simulink model "Assembly_Throwing_Arm"  (R2021a)
settings: Solver=ode15s  StartTime=0.0  StopTime=0.09
InitFcn:
  | contact_stiffness = 2000;
  | contact_damping = 10;
  | 
  | %% Parameters
  | 
  | %------------------- Mechanical -------------------%
  | arm_len = 0.106;
  | launch_ang = 45*(pi/180);
  | th_start = 0;
  | r_ball = 31.5/1000;
  | g = -9.80665;
  | 
  | %------------------- Electrical -------------------%
  | R = 0.194;
  | L = 0.097*1e-3;
  | K_m = 1/24.48;
  | V_max = 24;
  | neta = 0.70;
  | n = 6.5;
  | f_s = 4000;
  | NL_speed = 1200;
  | R_speed = 1050;
  | R_power = 240;
  | NL_current = 0.98;
  | 
  | 
  | %NL_speed = 589;
  | %R_speed = 469;
  | %R_power = 24*15.7;
  | %NL_current = 0.98;
model workspace: external: MATLAB File C:\Users\Imad\Downloads\Throwing Arm 3\Assembly_Throwing_Arm_DataFile.m (data not in the file)
values from neighbouring files (symbols this model uses):
  smiData = struct    [Assembly_Throwing_Arm_DataFile.m]
  target = target_given(1,3)    [Script_Throwing_Arm.m]
undefined symbols (not defined in the file or in its folder): X, Y, Z
libraries: sm_lib x20, nesl_utility x9, fl_lib x8, ee_lib x3, pid_lib x2
(part 1 of 2)
settings Model: OrderedModelArguments=off  Creator=Imad  LastModifiedBy=Imad
settings SolverCC: ZeroCrossControl=DisableAll

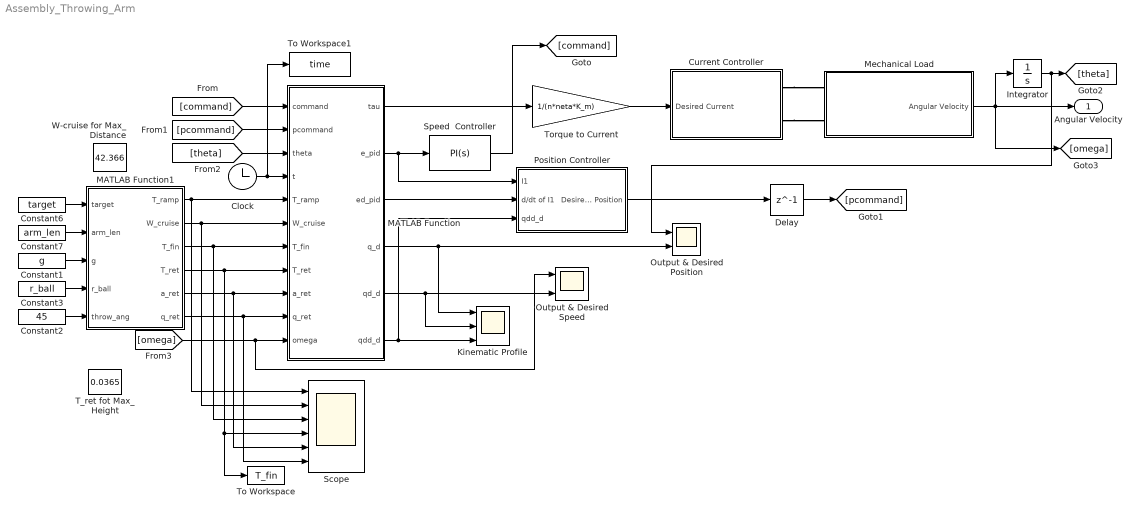
== system Assembly_Throwing_Arm ==
  Clock : Clock
  Constant1 : Constant  Value=g
  Constant2 : Constant  Value=45
  Constant3 : Constant  Value=r_ball
  Constant6 : Constant  Value=target
  Constant7 : Constant  Value=arm_len
  Current Controller : Subsystem
  Delay : Delay  DelayLength=1  SampleTime=1/(1*f_s)
  Integrator : Integrator
  Kinematic Profile : Scope  NumInputPorts=3
  MATLAB Function : MATLAB Function  TreatAsAtomicUnit=on
  MATLAB Function1 : MATLAB Function  TreatAsAtomicUnit=on
  Mechanical Load : Subsystem
  Output & Desired Position : Scope  NumInputPorts=2
  Output & Desired Speed : Scope  NumInputPorts=2
  "Position Controller " : Subsystem
  Scope : Scope  NumInputPorts=6
  Speed  Controller : pid_lib/PID Controller  Controller=PI  Form=Parallel  TimeDomain=Continuous-time  UseExternalTs=off  SampleTime=1/4000  IntegratorMethod=Forward Euler  FilterMethod=Forward Euler  ControllerParametersSource=internal  P=970*L*9  I=135*R  D=-0.5  UseFilter=on  N=100  TunerSelectOption=Frequency Response Based  InitialConditionSource=internal  InitialConditionForIntegrator=0  InitialConditionForFilter=0  DifferentiatorICPrevScaledInput=0  ExternalReset=none  TrackingMode=off  Kt=1  LimitOutput=off  SatLimitsSource=internal  UpperSaturationLimit=inf  LowerSaturationLimit=-inf  LinearizeAsGain=on  AntiWindupMode=none  Kb=1  POutMin=[]  POutMax=[]  IOutMin=[]  IOutMax=[]  DOutMin=[]  DOutMax=[]  NOutMin=[]  NOutMax=[]  SumOutMin=[]  SumOutMax=[]  SaturationOutMin=[]  SaturationOutMax=[]  PParamMin=[]  PParamMax=[]  IParamMin=[]  IParamMax=[]  DParamMin=[]  DParamMax=[]  NParamMin=[]  NParamMax=[]  KbParamMin=[]  KbParamMax=[]  KtParamMin=[]  KtParamMax=[]  KbOutMin=[]  KbOutMax=[]  KtOutMin=[]  KtOutMax=[]  IntegratorOutMin=[]  IntegratorOutMax=[]  FilterOutMin=[]  FilterOutMax=[]  SumI1OutMin=[]  SumI1OutMax=[]  SumI2OutMin=[]  SumI2OutMax=[]  SumI3OutMin=[]  SumI3OutMax=[]  SumI4OutMin=[]  SumI4OutMax=[]  SumDOutMin=[]  SumDOutMax=[]  DifferentiatorOutMin=[]  DifferentiatorOutMax=[]  FilterDiffOutCoefMin=[]  FilterDiffOutCoefMax=[]  ReciprocalOutMin=[]  ReciprocalOutMax=[]  SumDenOutMin=[]  SumDenOutMax=[]  SumNumOutMin=[]  SumNumOutMax=[]  DivideOutMin=[]  DivideOutMax=[]  UdiffTsProdOutMin=[]  UdiffTsProdOutMax=[]  NTsProdOutMin=[]  NTsProdOutMax=[]  UintegralTsProdOutMin=[]  UintegralTsProdOutMax=[]  UngainTsProdOutMin=[]  UngainTsProdOutMax=[]  IntegratorContinuousStateAttributes=''  IntegratorStateMustResolveToSignalObject=off  IntegratorRTWStateStorageClass=Auto  FilterContinuousStateAttributes=''  FilterStateMustResolveToSignalObject=off  FilterRTWStateStorageClass=Auto  ParallelPVariant=InternalParameters  IdealPVariant=Disabled  IVariant=InternalParameters  DVariant=Disabled  IntegratorVariant=Continuous  SatVariant=Disabled  AWVariant=Passthrough  PCopyVariant=Disabled  TRVariant=Disabled  FdbkBlocksVariant=Forward  IdealPFdbkVariant=Disabled  SatFdbkVariant=Disabled  DerivativeFilterVariant=Disabled  NVariant=Disabled  NCopyVariant=Disabled_SignalSpec  FilterICVariant=Disabled  IntegratorICVariant=InternalICs  ExternalResetVariant=Disabled  TRSumVariant=Passthrough  SumFdbkVariant=Disabled  SumVariant=Sum_PI  TsampFilterVariant=InternalTs  TsampNgainVariant=Passthrough  TsampIntegralVariant=Passthrough  ExternalSaturationOutDataTypeStr=Inherit: Same as second input
  T_ret fot Max_Height : Constant  Value=0.0365
  To Workspace : ToWorkspace  VariableName=T_fin  SampleTime=-1
      settings: Save2DSignal=2-D array (concatenate along first dimension)
  To Workspace1 : ToWorkspace  VariableName=time  SampleTime=-1
  Torque to Current : Gain  Gain=1/(n*neta*K_m)
  W-cruise for Max_Distance : Constant  Value=42.366
  Angular Velocity : Outport
  wires:
  MATLAB Function/3(ed_pid) -> "Position Controller "/2(d/dt of I1)
  MATLAB Function/6(qdd_d) -> Kinematic Profile/3, "Position Controller "/3(qdd_d)
  Clock/1 -> To Workspace1/1, MATLAB Function/4(t)
  [command] -> MATLAB Function/1(command)
  [pcommand] -> MATLAB Function/2(pcommand)
  Torque to Current/1 -> Current Controller/1("Desired Current ")
  Mechanical Load/1(Angular Velocity) -> Integrator/1, Angular Velocity/1, [omega]
  Delay/1 -> [pcommand]
  [theta] -> MATLAB Function/3(theta)
  Speed  Controller/1 -> [command]
  MATLAB Function1/1(T_ramp) -> Scope/1, MATLAB Function/5(T_ramp)
  MATLAB Function1/2(W_cruise) -> MATLAB Function/6(W_cruise), Scope/2
  MATLAB Function1/3(T_fin) -> Scope/3, MATLAB Function/7(T_fin)
  MATLAB Function1/4(T_ret) -> MATLAB Function/8(T_ret), Scope/4, To Workspace/1
  MATLAB Function/2(e_pid) -> Speed  Controller/1, "Position Controller "/1(I1)
  Constant7/1 -> MATLAB Function1/2(arm_len)
  Constant6/1 -> MATLAB Function1/1(target)
  Constant2/1 -> MATLAB Function1/5(throw_ang)
  Constant1/1 -> MATLAB Function1/3(g)
  MATLAB Function1/5(a_ret) -> MATLAB Function/9(a_ret), Scope/5
  MATLAB Function1/6(q_ret) -> MATLAB Function/10(q_ret), Scope/6
  "Position Controller "/1(Desired Position) -> Delay/1
  MATLAB Function/1(tau) -> Torque to Current/1
  Constant3/1 -> MATLAB Function1/4(r_ball)
  Integrator/1 -> Output & Desired Position/1, [theta]
  MATLAB Function/4(q_d) -> Output & Desired Position/2, Kinematic Profile/1
  [omega] -> Output & Desired Speed/1, MATLAB Function/11(omega)
  MATLAB Function/5(qd_d) -> Output & Desired Speed/2, Kinematic Profile/2
  connections:
  Current Controller/RConn1 -- Mechanical Load/LConn1
  Current Controller/RConn2 -- Mechanical Load/LConn2

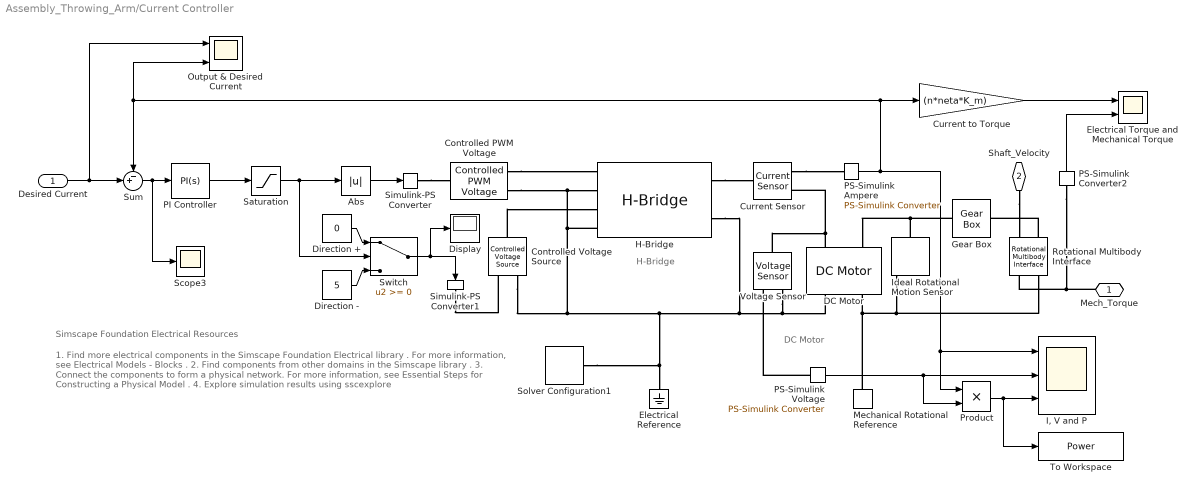
== system Assembly_Throwing_Arm/Current Controller ==
  note: H-Bridge
  note: DC Motor
  note: 1. Find more electrical components in the Simscape Foundation Electrical library .
      | For more information, see Electrical Models - Blocks .
      | 2. Find components from other domains in the Simscape library .
      | 3. Connect the components to form a physical network.
      | For more information, see Essential Steps for Constructing a Physical Model .
      | 4. Explore simulation results using sscexplore
  note: Simscape Foundation Electrical Resources
  "Desired Current " : Inport
  Abs : Abs
  Controlled PWM Voltage : ee_lib/Integrated Circuits/Controlled PWM Voltage  F=f_s Hz  TD=0 s  pulse_width_offset=0 s  pulse_min=1 us  Vmin=0 V  Vmax=12 V  Vm=V_max V  pwm_or_av=2  event_type=1  sample_time=1e-6 s  u_min=0  u_max=V_max
      settings: InternalSimscapePortConfiguration="{\"Bottom\":[],\"Left\":[{\"id\":\"u\",\"label\":\"u\",\"type\":\"input\"}],\"Right\":[{\"id\":\"p2\",\"label\":\"PWM\",\"type\":\"foundation.electrical.electrical\"},{\"id\":\"n2\",\"label\":\"REF\",\"type\":\"foundation.electrical.electrical\"}],\"Top\":[]}"
  Controlled Voltage Source : fl_lib/Electrical/Electrical Sources/Controlled Voltage Source
  Current Sensor : fl_lib/Electrical/Electrical Sensors/Current Sensor
  Current to Torque : Gain  Gain=(n*neta*K_m)
  DC Motor : ee_lib/Electromechanical/Brushed Motors/DC Motor  field_option=ee.enum.field_option.pm  Rf=100 Ohm  Lf=1 H  Laf=0.15 H  If0=0 A  parameterization=ee.enum.dcparam_option.load_speed  Ra=R Ohm  La=L H  emf_or_torque=ee.enum.emf_or_torque.kv  Kv=K_m V/rpm  Ki=6.876e-4 N*m/A  T_stall=4.5 N*m  w_max=NL_speed rpm  w_rated=R_speed rpm  P_rated=R_power W  V_rated=V_max V  J=2000 g*cm^2  lam_param=ee.enum.lam_param.current  lam=(1.114e-4) N*m/(rad/s)  i_noload=NL_current A  V_i_noload=V_max V  speed0=0 rpm  enable_fault_armature=ee.enum.faults.faultEnable.no  rev_faulted=1 / 3  G_faulted_armature=1e-5 S  fault_trigger_armature=ee.enum.faults.faultTrigger.temporal  t_fault_armature=1 s  max_permissible_current_armature=inf A  t_fail_on_current_armature=1 s  enable_fault_field=ee.enum.faults.faultEnable.no  G_faulted_field=1e-5 S  fault_trigger_field=ee.enum.faults.faultTrigger.temporal  t_fault_field=1 s  max_permissible_current_field=inf A  t_fail_on_current_field=1 s  fault_action=ee.enum.faults.faultAction.none  alpha=3.93e-3 1/K  Tmeas=25 degC  thermal_mass=100 J/K  initial_temperature=25 degC
  Direction + : Constant  Value=0
  Direction - : Constant  Value=5
  Display : Display
  Electrical Reference : fl_lib/Electrical/Electrical Elements/Electrical Reference
  Electrical Torque and Mechanical Torque : Scope  NumInputPorts=2
  Gear Box : fl_lib/Mechanical/Mechanisms/Gear Box  ratio=1  t_in_specify=off  t_in_priority=None  t_in=0 N*m  t_in_nominal_specify=off  t_in_nominal_unit=N*m  t_in_nominal_value=1  t_out_specify=off  t_out_priority=None  t_out=0 N*m  t_out_nominal_specify=off  t_out_nominal_unit=N*m  t_out_nominal_value=1
      settings: LogSimulationData=on
  H-Bridge : ee_lib/Semiconductors & Converters/Converters/H-Bridge  supply_ports=ee.enum.supply_ports.hidesupply  Venable=2 V  Vmax=V_max V  Vreverse=2.5 V  Vbrake=2.5 V  Vm=V_max V  pwm_or_av=ee.enum.pwm_or_av.averaged  regenerative_braking_mode=ee.enum.converters.regenerative_braking_mode.always_enabled  discontinuous=ee.enum.current_profile.continuous  freewheeling_mode=ee.enum.converters.freewheeling_mode.two_diodes  Ron=0.55 Ohm  Don=1.3/3 Ohm  Goff=1e-6 S  Rload=10 Ohm  Lload=1e-5 H  F=10 kHz  thermal_mass=(1.25/298.15)*5 J/K  initial_temperature=298.15 K  Ron2=0.9 Ohm  Don2=1.7/3 Ohm  Tmeas=298.15 K  Tmeas2=360.65 K
  "I, V and P" : Scope  NumInputPorts=3
  Ideal Rotational Motion Sensor : fl_lib/Mechanical/Mechanical Sensors/Ideal Rotational Motion Sensor  wrap_angle=simscape.enum.onoff.off  offset=0 rad
  Mechanical Rotational Reference : fl_lib/Mechanical/Rotational Elements/Mechanical Rotational Reference
  Output & Desired Current : Scope  NumInputPorts=2
  PI Controller : pid_lib/PID Controller  Controller=PI  Form=Parallel  TimeDomain=Continuous-time  UseExternalTs=off  SampleTime=1/4000  IntegratorMethod=Forward Euler  FilterMethod=Forward Euler  ControllerParametersSource=internal  P=1200*L  I=10000*R  D=0.1  UseFilter=on  N=100  TunerSelectOption=Transfer Function Based (PID Tuner App)  ZeroCross=off  InitialConditionSource=internal  InitialConditionForIntegrator=0  InitialConditionForFilter=0  DifferentiatorICPrevScaledInput=0  ExternalReset=none  TrackingMode=off  Kt=1  LimitOutput=off  SatLimitsSource=internal  UpperSaturationLimit=inf  LowerSaturationLimit=-inf  LinearizeAsGain=on  AntiWindupMode=none  Kb=1  POutMin=[]  POutMax=[]  IOutMin=[]  IOutMax=[]  DOutMin=[]  DOutMax=[]  NOutMin=[]  NOutMax=[]  SumOutMin=[]  SumOutMax=[]  SaturationOutMin=[]  SaturationOutMax=[]  PParamMin=[]  PParamMax=[]  IParamMin=[]  IParamMax=[]  DParamMin=[]  DParamMax=[]  NParamMin=[]  NParamMax=[]  KbParamMin=[]  KbParamMax=[]  KtParamMin=[]  KtParamMax=[]  KbOutMin=[]  KbOutMax=[]  KtOutMin=[]  KtOutMax=[]  IntegratorOutMin=[]  IntegratorOutMax=[]  FilterOutMin=[]  FilterOutMax=[]  SumI1OutMin=[]  SumI1OutMax=[]  SumI2OutMin=[]  SumI2OutMax=[]  SumI3OutMin=[]  SumI3OutMax=[]  SumI4OutMin=[]  SumI4OutMax=[]  SumDOutMin=[]  SumDOutMax=[]  DifferentiatorOutMin=[]  DifferentiatorOutMax=[]  FilterDiffOutCoefMin=[]  FilterDiffOutCoefMax=[]  ReciprocalOutMin=[]  ReciprocalOutMax=[]  SumDenOutMin=[]  SumDenOutMax=[]  SumNumOutMin=[]  SumNumOutMax=[]  DivideOutMin=[]  DivideOutMax=[]  UdiffTsProdOutMin=[]  UdiffTsProdOutMax=[]  NTsProdOutMin=[]  NTsProdOutMax=[]  UintegralTsProdOutMin=[]  UintegralTsProdOutMax=[]  UngainTsProdOutMin=[]  UngainTsProdOutMax=[]  IntegratorContinuousStateAttributes=''  IntegratorStateMustResolveToSignalObject=off  IntegratorRTWStateStorageClass=Auto  FilterContinuousStateAttributes=''  FilterStateMustResolveToSignalObject=off  FilterRTWStateStorageClass=Auto  ParallelPVariant=InternalParameters  IdealPVariant=Disabled  IVariant=InternalParameters  DVariant=Disabled  IntegratorVariant=Continuous  SatVariant=Disabled  AWVariant=Passthrough  PCopyVariant=Disabled  TRVariant=Disabled  FdbkBlocksVariant=Forward  IdealPFdbkVariant=Disabled  SatFdbkVariant=Disabled  DerivativeFilterVariant=Disabled  NVariant=Disabled  NCopyVariant=Disabled_SignalSpec  FilterICVariant=Disabled  IntegratorICVariant=InternalICs  ExternalResetVariant=Disabled  TRSumVariant=Passthrough  SumFdbkVariant=Disabled  SumVariant=Sum_PI  TsampFilterVariant=InternalTs  TsampNgainVariant=Passthrough  TsampIntegralVariant=Passthrough  ExternalSaturationOutDataTypeStr=Inherit: Same as second input
  PS-Simulink Ampere : nesl_utility/PS-Simulink Converter  PhysicalDomain=network_engine_domain  SubClassName=ps_output  LeftPortType=input  RightPortType=output  PseudoPeriodic=off  Frequencies=[]  Unit=A  AffineConversion=off
      settings: SourceProductBaseCode=PW,SS
  PS-Simulink Converter2 : nesl_utility/PS-Simulink Converter  PhysicalDomain=network_engine_domain  SubClassName=ps_output  LeftPortType=input  RightPortType=output  PseudoPeriodic=off  Frequencies=[]  Unit=inherit  AffineConversion=off
      settings: SourceProductBaseCode=PW,SS
  PS-Simulink Voltage : nesl_utility/PS-Simulink Converter  PhysicalDomain=network_engine_domain  SubClassName=ps_output  LeftPortType=input  RightPortType=output  PseudoPeriodic=off  Frequencies=[]  Unit=V  AffineConversion=off
      settings: SourceProductBaseCode=PW,SS
  Product : Product
  Rotational Multibody Interface : fl_lib/Mechanical/Multibody Interfaces/Rotational Multibody Interface
      settings: SourceProductBaseCode=SS
  Saturation : Saturate  UpperLimit=V_max  LowerLimit=-V_max
  Scope3 : Scope
  Simulink-PS Converter : nesl_utility/Simulink-PS Converter  PhysicalDomain=network_engine_domain  SubClassName=ps_input  LeftPortType=input  RightPortType=output  PseudoPeriodic=off  Frequencies=[]  NoiseDistribution=none  NoiseParameters=[]  Unit=1  AffineConversion=off  FilteringAndDerivatives=provide  SimscapeFilterOrder=1  InputFilterTimeConstant=0.001  UdotUserProvided=0
      settings: SourceProductBaseCode=PW,SS
  Simulink-PS Converter1 : nesl_utility/Simulink-PS Converter  PhysicalDomain=network_engine_domain  SubClassName=ps_input  LeftPortType=input  RightPortType=output  PseudoPeriodic=off  Frequencies=[]  NoiseDistribution=none  NoiseParameters=[]  Unit=1  AffineConversion=off  FilteringAndDerivatives=provide  SimscapeFilterOrder=1  InputFilterTimeConstant=0.001  UdotUserProvided=0
      settings: SourceProductBaseCode=PW,SS
  Solver Configuration1 : nesl_utility/Solver Configuration  PhysicalDomain=network_engine_domain  SubClassName=solver  LeftPortType=input  RightPortType=generic  Tones=[]  Harmonics=[]  SimulateNoise=off  Profile=off  UseLocalSampling=off  EnableSwitchedLinearOptims=on  FrequencyDomain=off  UseCCode=off  RelTol=0.001  AbsTol=1e-06  MinStep=1e-09  ToWorkspace=off  RevertToSquareIcSolve=off  NumHomotopyIterations=100  PhasorMode=off  PhasorModeNumHarmonics=1  DoDC=off  ResidualTolerance=1e-09  UseLocalSolver=off  LocalSolverChoice=NE_BACKWARD_EULER_ADVANCER  LocalSolverSampleTime=0.001  DoFixedCost=off  MaxNonlinIter=3  MaxModeIter=2  ComputeImpulses=off  ImpulseIterations=2  LinearAlgebra=auto  EquationFormulation=NE_TIME_EF  DelaysMemoryBudget=1024  AutomaticFiltering=on  FilteringTimeConstant=0.001  PartitionStorageMethod=AS_NEEDED  PartitionMemoryBudget=1024  PartitionMethod=ROBUST
      settings: SourceProductBaseCode=PW,SS
  Sum : Sum  Inputs=-+|
  Switch : Switch
  To Workspace : ToWorkspace  VariableName=Power  SampleTime=-1
  Voltage Sensor : fl_lib/Electrical/Electrical Sensors/Voltage Sensor
  Mech_Torque : PMIOPort  Side=Right
  Shaft_Velocity : PMIOPort  Port=2  Side=Right
  wires:
  PS-Simulink Voltage/1 -> "I, V and P"/2, Product/2
  Switch/1 -> Display/1, Simulink-PS Converter1/1
  Sum/1 -> PI Controller/1, Scope3/1
  Current to Torque/1 -> Electrical Torque and Mechanical Torque/1
  Direction +/1 -> Switch/1
  Direction -/1 -> Switch/3
  PI Controller/1 -> Saturation/1
  PS-Simulink Converter2/1 -> Electrical Torque and Mechanical Torque/2
  Saturation/1 -> Abs/1, Switch/2
  Abs/1 -> Simulink-PS Converter/1
  "Desired Current "/1 -> Output & Desired Current/1, Sum/2
  PS-Simulink Ampere/1 -> Output & Desired Current/2, Sum/1, Current to Torque/1, Product/1, "I, V and P"/1
  Product/1 -> "I, V and P"/3, To Workspace/1
  connections:
  PS-Simulink Voltage/LConn1 -- Voltage Sensor/RConn1
  Simulink-PS Converter/RConn1 -- Controlled PWM Voltage/LConn1
  Controlled Voltage Source/LConn1 -- H-Bridge/LConn3
  H-Bridge/RConn1 -- Current Sensor/LConn1
  Controlled PWM Voltage/RConn1 -- H-Bridge/LConn1
  DC Motor/LConn1 -- Voltage Sensor/LConn1 -- Current Sensor/RConn2
  DC Motor/RConn2 -- Rotational Multibody Interface/LConn2 -- Ideal Rotational Motion Sensor/RConn1 -- Mechanical Rotational Reference/LConn1
  Current Sensor/RConn1 -- PS-Simulink Ampere/LConn1
  H-Bridge/RConn2 -- Solver Configuration1/RConn1 -- Electrical Reference/LConn1 -- H-Bridge/LConn4 -- Controlled PWM Voltage/RConn2 -- H-Bridge/LConn2 -- Controlled Voltage Source/RConn2 -- DC Motor/RConn1 -- Voltage Sensor/RConn2
  Simulink-PS Converter1/RConn1 -- Controlled Voltage Source/RConn1
  Ideal Rotational Motion Sensor/LConn1 -- Gear Box/LConn1 -- DC Motor/LConn2
  PS-Simulink Converter2/LConn1 -- Rotational Multibody Interface/LConn1 -- Mech_Torque/RConn1
  Rotational Multibody Interface/RConn2 -- Gear Box/RConn1
  Shaft_Velocity/RConn1 -- Rotational Multibody Interface/RConn1
